simulink model "RST_final"  (R2022b)
settings: Solver=VariableStepAuto  StartTime=0.0  StopTime=50  RelTol=1e-3
values from neighbouring files (symbols this model uses):
  A = [1 -0.9535]    [script_proiect.m]
  A1 = H_impusd.den{1}    [script_proiect.m]
  B = 0.05394    [script_proiect.m]
  B1 = H_impusd.num{1}    [script_proiect.m]
  R = [pol(7:8)]'    [script_proiect.m]
  S = conv(S1,[1 -1])    [script_proiect.m]
  T = H_impusd.den{1}/ sum(B)    [script_proiect.m]
settings Model: Creator=gabri  LastModifiedBy=Ioana-Roxana

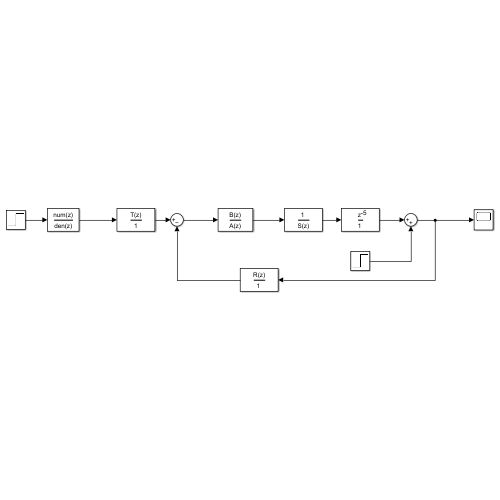
[thumbnail: Simulink's stored preview of the top-level diagram]
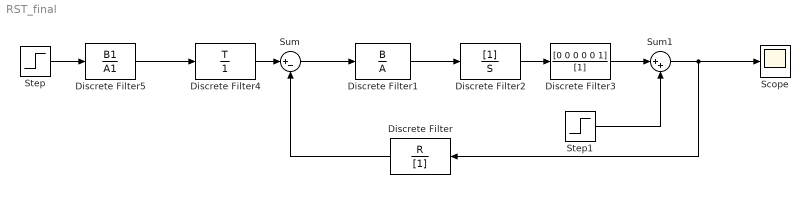
== system RST_final ==
  Discrete Filter : DiscreteFilter  Numerator=R  Denominator=[1]  SampleTime=0.1
  Discrete Filter1 : DiscreteFilter  Numerator=B  Denominator=A  SampleTime=0.1
  Discrete Filter2 : DiscreteFilter  Denominator=S  SampleTime=0.1
  Discrete Filter3 : DiscreteFilter  Numerator=[0 0 0 0 0 1]  Denominator=[1]  SampleTime=0.1
  Discrete Filter4 : DiscreteFilter  Numerator=T  Denominator=1  SampleTime=0.1
  Discrete Filter5 : DiscreteFilter  Numerator=B1  Denominator=A1  SampleTime=0.1
  Scope : Scope
  Step : Step  After=120  SampleTime=0.1
  Step1 : Step  Time=10  After=20  SampleTime=0.1
  Sum : Sum  Inputs=|+-
  Sum1 : Sum  Inputs=|++
  wires:
  Step1/1 -> Sum1/2
  Sum1/1 -> Discrete Filter/1, Scope/1
  Discrete Filter/1 -> Sum/2
  Discrete Filter3/1 -> Sum1/1
  Step/1 -> Discrete Filter5/1
  Discrete Filter2/1 -> Discrete Filter3/1
  Discrete Filter1/1 -> Discrete Filter2/1
  Sum/1 -> Discrete Filter1/1
  Discrete Filter5/1 -> Discrete Filter4/1
  Discrete Filter4/1 -> Sum/1
